simulink model "MPC_sim"  (R2023b)
settings: Solver=VariableStepAuto  StartTime=0.0  StopTime=10.0  RelTol=1e-3
values from neighbouring files (symbols this model uses):
  Lc = theta(6, 1)    [lin_MPC.m]
  Rtot = theta(5, 1)    [lin_MPC.m]
settings Model: Creator=lollo  LastModifiedBy=lollo
settings DataIOCC: SaveFormat=StructureWithTime

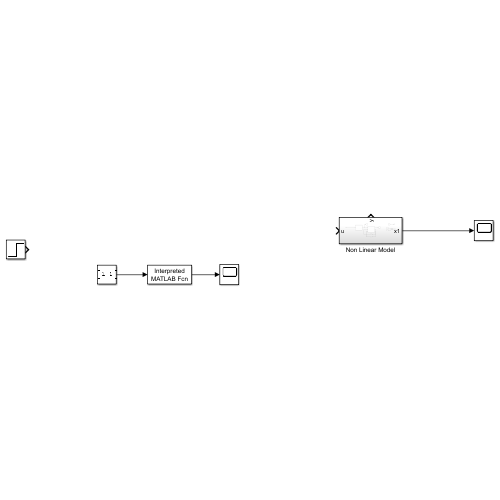
[thumbnail: Simulink's stored preview of the top-level diagram]
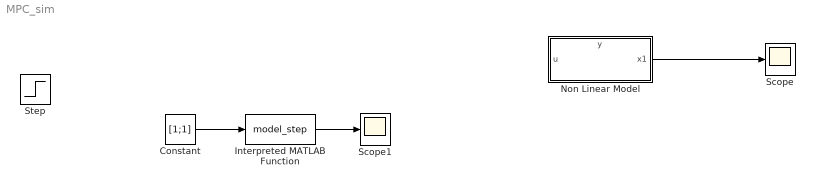
== system MPC_sim ==
  Constant : Constant  Value=[1;1]
  Interpreted MATLAB Function : MATLABFcn  MATLABFcn=model_step
  Non Linear Model : Subsystem
      settings: PortSchema="{\"entries\":[{\"content\":{\"sides\":[{\"content\":{\"connectorIds\":[\"In1\"]},\"type\":\"ConnectorPlacement.EquallySpacedRectSide\",\"uuid\":\"5ca3b90f-5d3c-4aa5-a900-af453f2fdae0\"},{\"content\":{\"connectorIds\":[\"Out1\"],\"side\":\"RIGHT\"},\"type\":\"ConnectorPlacement.EquallySpacedRectSide\",\"uuid\":\"52db600d-e1b5-431e-8054-3c8f4eef190e\"},{\"content\":{\"connectorIds\":[\"Out2\"],\"side\":\"TOP\"},\"type\":\"ConnectorPlacement.EquallySpacedRectSide\",\"uuid\":\"16d45e1c-4ef0-4ebe-8fe1-04ddeb9dc0f3\"}]},\"type\":\"ConnectorPlacement.EquallySpacedConnector\",\"uuid\":\"771bde15-64e9-44eb-bf14-659d8ae18ddd\"}],\"packageUris\":[\"http://schema.mathworks.com/mf0/Connector/R2020b\"],\"version\":\"1.0\"}"
  Scope : Scope
  Scope1 : Scope
  Step : Step  After=0.001  SampleTime=0
  wires:
  Non Linear Model/1(x1) -> Scope/1
  Constant/1 -> Interpreted MATLAB Function/1
  Interpreted MATLAB Function/1 -> Scope1/1

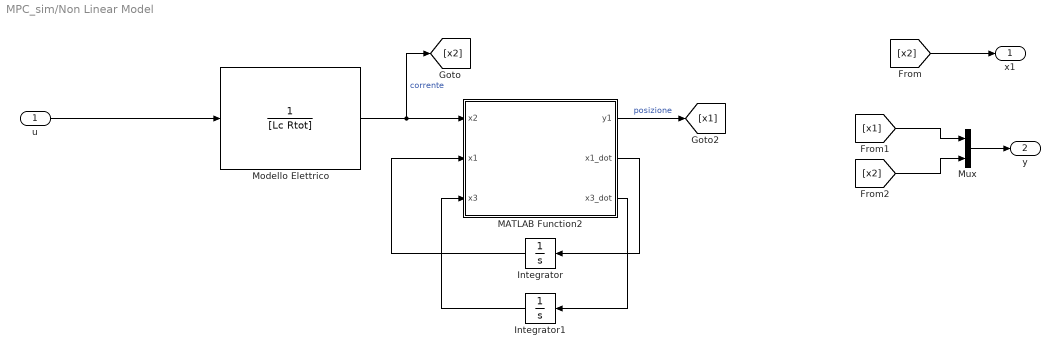
== system MPC_sim/Non Linear Model ==
  u : Inport
  Integrator : Integrator
  Integrator1 : Integrator
  MATLAB Function2 : MATLAB Function  TreatAsAtomicUnit=on
  Modello Elettrico : TransferFcn  Denominator=[Lc Rtot]
  Mux : Mux  Inputs=2
  x1 : Outport
  y : Outport  Port=2
  wires:
  MATLAB Function2/1(y1) -> [x1]  "posizione"
  MATLAB Function2/2(x1_dot) -> Integrator/1
  Integrator/1 -> MATLAB Function2/2(x1)
  MATLAB Function2/3(x3_dot) -> Integrator1/1
  Integrator1/1 -> MATLAB Function2/3(x3)
  Modello Elettrico/1 -> [x2], MATLAB Function2/1(x2)  "corrente"
  u/1 -> Modello Elettrico/1
  [x2] -> x1/1
  Mux/1 -> y/1
  [x1] -> Mux/1
  [x2] -> Mux/2

== matlab function MPC_sim/Non Linear Model/MATLAB Function2 ==
  data: y1 output; x2 input; x1_dot output; x1 input; x3 input; x3_dot output
function [y1,x1_dot, x3_dot] = fcn(x2, x1, x3)
    m = 0.0657;
    g = 9.81;
    k_mag = 2.4405e-05;
    Rtot = 9.7585;
    Lc = 0.3708;
    y0 = 0.012;
    
    x1_dot = x3;
    if x1 < y0
        x3_dot = (k_mag/m)*(x2/(y0-x1))^2 - g;
    else
        x1 = 0.012;
        x3_dot = 0;
        x3 = 0;
    end

    
    % condizioni
    if x1 <=0 && x3_dot < 0
        x1 = 0;
        x3 = 0;
        x3_dot = 0;
    end
y1 = x1;
